simulink model "sldemo_state_logging2"  (Simulink 7.6)
settings: Solver=ode1  StartTime=0.0  StopTime=10.0  FixedStep=0.1  RelTol=1e-3
settings Model: Creator=The MathWorks Inc.  ExtModeAutoUpdateStatusClock=off
settings DataIOCC: LimitDataPoints=off  SaveOutput=off  SaveState=on  SignalLogging=off
settings OptimizationCC: InitFltsAndDblsToZero=on
settings DebuggingCC: SaveWithParameterizedLinksMsg=none  SignalResolutionControl=TryResolveAllWithWarning  MultiTaskDSMMsg=warning  MultiTaskCondExecSysMsg=none
settings RTWCC: IncludeERTFirstTime=on
settings GRTTargetCC: TargetFcnLib=ansi_tfl_tmw.mat

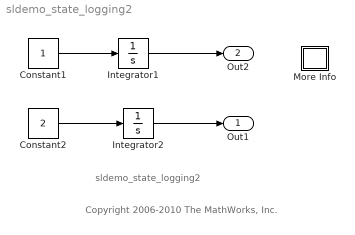
== system sldemo_state_logging2 ==
  note: sldemo_state_logging2
  note: Copyright 2006-2010 The MathWorks, Inc.
  Constant1 : Constant
  Constant2 : Constant  Value=2
  Integrator1 : Integrator
  Integrator2 : Integrator
  More Info : Subsystem
      settings: OpenFcn=showdemo('sldemo_state_logging_script')
      mask Display: disp('?')
  Out1 : Outport
  Out2 : Outport  Port=2
  wires:
  Constant2/1 -> Integrator2/1
  Constant1/1 -> Integrator1/1
  Integrator2/1 -> Out1/1
  Integrator1/1 -> Out2/1

== system sldemo_state_logging2/More Info ==
